simulink model "SimulateAppliancePower"  (R2021a)
settings: Solver=ode45  StartTime=0  StopTime=5419320  RelTol=1e-3
settings Model: Creator=pankaja  LastModifiedBy=pankaja
settings DataIOCC: SaveFormat=StructureWithTime

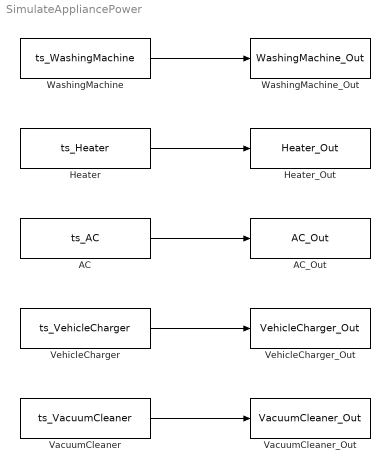
== system SimulateAppliancePower ==
  AC : FromWorkspace  VariableName=ts_AC  SampleTime=-1
  AC_Out : ToWorkspace  VariableName=AC_Out  SaveFormat=Structure With Time  SampleTime=-1
  Heater : FromWorkspace  VariableName=ts_Heater  SampleTime=-1
  Heater_Out : ToWorkspace  VariableName=Heater_Out  SaveFormat=Structure With Time  SampleTime=-1
  VacuumCleaner : FromWorkspace  VariableName=ts_VacuumCleaner  SampleTime=-1
  VacuumCleaner_Out : ToWorkspace  VariableName=VacuumCleaner_Out  SaveFormat=Structure With Time  SampleTime=-1
  VehicleCharger : FromWorkspace  VariableName=ts_VehicleCharger  SampleTime=-1
  VehicleCharger_Out : ToWorkspace  VariableName=VehicleCharger_Out  SaveFormat=Structure With Time  SampleTime=-1
  WashingMachine : FromWorkspace  VariableName=ts_WashingMachine  SampleTime=-1
  WashingMachine_Out : ToWorkspace  VariableName=WashingMachine_Out  SaveFormat=Structure With Time  SampleTime=-1
  wires:
  WashingMachine/1 -> WashingMachine_Out/1
  Heater/1 -> Heater_Out/1
  AC/1 -> AC_Out/1
  VehicleCharger/1 -> VehicleCharger_Out/1
  VacuumCleaner/1 -> VacuumCleaner_Out/1
